simulink model "ex1_model"  (Simulink 9.1)
settings: Solver=VariableStepAuto  StartTime=0.0  StopTime=10  RelTol=1e-3
values from neighbouring files (symbols this model uses):
  B = [0;1;0;0;0;0]    [ECE21122L_3ECEC_Oliveros_JE_Expt3_4.m]    (also in ex1_parameter.m = 4; ex2_plots.m = 25; example1.m = [z;k/ai(1)]; mass_spring_a2.m = 0.5)
  K = 1    [ECE21122L_3ECEC_Oliveros_JE_Expt4_4.m]    (also in ECE21122L_3ECEC_Oliveros_JE_Expt6_A_9.m = -(s^4 + 12*s^3 + 41*s^2 + 30*s)/(s^2 + 5*s + 6); ECE21122L_3ECEC_Oliveros_JE_Expt6_B_9.m = -(s^2 + 2*s + 2)/(s^3 - 2*s + 4); ECE21122L_3ECEC_Oliveros_JE_Expt6_C_3.m = abs(1/(g*cg)); ECE21122L_3ECEC_Oliveros_JE_Expt7_B_3.m = 0.78)
  M = 2    [ex1_parameter.m]    (also in mass_spring_a2.m = 10)
settings Model: SuppressorTable=22 serialization::archive 11 0 6 0 0 0 0 0  Creator=jillianeuniceb.oliveros  LastModifiedBy=jillianeuniceb.oliveros
settings DataIOCC: SaveFormat=Dataset
settings OptimizationCC: LifeSpan=auto
settings DebuggingCC: UnderspecifiedInitializationDetection=Simplified  MergeDetectMultiDrivingBlocksExec=error  SFUnexpectedBacktrackingDiag=error  SFNoUnconditionalDefaultTransitionDiag=error  SFExecutionAtInitializationDiag=warning
settings HardwareCC: ProdBitPerPointer=64  ProdBitPerSizeT=64  ProdBitPerPtrDiffT=64  ProdLargestAtomicFloat=Float  ProdIntDivRoundTo=Zero  ProdEndianess=LittleEndian  ProdWordSize=64  ProdHWDeviceType=Intel->x86-64 (Windows64)
settings ModelReferenceCC: PropagateSignalLabelsOutOfModel=on
settings CodeAppCC: StateflowObjectComments=off
settings GRTTargetCC: TargetLangStandard=C99 (ISO)  CombineOutputUpdateFcns=on  GRTInterface=off
settings ConfigComp: CovMetricSettings=dwe  CovHtmlReporting=off  CovSaveCumulativeToWorkspaceVar=off  CovSaveSingleToWorkspaceVar=off  CovExternalEMLEnable=on

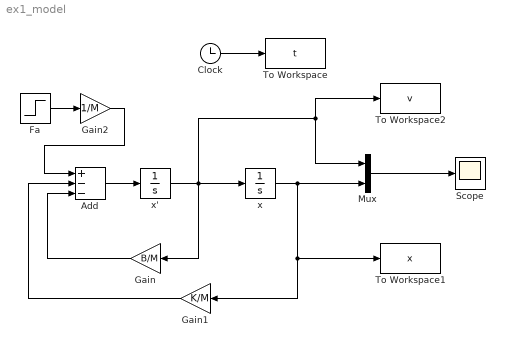
== system ex1_model ==
  Add : Sum  Inputs=+--
  Clock : Clock
  Fa : Step  After=8  SampleTime=0
  Gain : Gain  Gain=B/M
  Gain1 : Gain  Gain=K/M
  Gain2 : Gain  Gain=1/M
  Mux : Mux  Inputs=2
  Scope : Scope
  To Workspace : ToWorkspace  VariableName=t  SampleTime=-1
  To Workspace1 : ToWorkspace  VariableName=x  SampleTime=-1
  To Workspace2 : ToWorkspace  VariableName=v  SampleTime=-1
  x : Integrator
  x' : Integrator
  wires:
  Add/1 -> x'/1
  Gain2/1 -> Add/1
  Gain1/1 -> Add/2
  Gain/1 -> Add/3
  x/1 -> To Workspace1/1, Gain1/1, Mux/2
  Mux/1 -> Scope/1
  Fa/1 -> Gain2/1
  Clock/1 -> To Workspace/1
  x'/1 -> Gain/1, x/1, Mux/1, To Workspace2/1
